simulink model "ImSimulazione"  (Simulink 8.7)
settings: Solver=ode45  StartTime=0.0  StopTime=t(end)+Tf  FixedStep=Tf  RelTol=1e-3
PreLoadFcn:
  | initFunction
InitFcn:
  | initFunctionIm
StopFcn:
  | figure
  | subplot(31,1)
  | plot(err_q.data(1:50))
  | subplot(312)
  | plot(err_dq.data(1:50))
  | subplot(313)
  | plot(err_ddq.data(1:50))
values from neighbouring files (symbols this model uses):
  FM = Kr^-1*Fv*Kr^-1    [ControlloreUnico.m]    (also in SimulazioneLsim.m = Kr^-1*Fv_att*Kr^-1; initFunction.m; initFunctionIm.m)
  Im = Kr^-1*Bconst*Kr^-1    [initFunction.m]    (also in initFunctionIm.m)
  KCA = diag([(-W(1,1)^2 + KM(1,1)*XR(1,1))/(KM(1,1)*KTA(1,1)*W(1,1)^2),             (-W(2,2)^2 + KM(2,2)*XR(2,2))/(KM(2,2)*KTA(2,2)*W(2,2)^2),             (-W(3,3)^2 + KM(3,3)*XR(3,3))/(KM(3,3)*KTA(3,3)*W(3,3)^2),             (-W(4,4)^2 + KM(4,4)*XR(4,4))/(KM(4,4)*KTA(4,4)*W(4,4)^2),             (-W(5,5)^2 + KM(5,5)*XR(5,5))/(KM(5,5)*KTA(5,5)*W(5,5)^2),             (-W(6,6)^2 + KM(6,6)*XR(6,6))/(KM(6,6)* ...(+20 chars)    [DesignControllersAcceleration_6.m]    (also in DesignControllersAcceleration_7.m; DiscreteControllersAcceleration_7.m)
  KM = Kv^-1    [DesignControllersAcceleration_6.m]    (also in DesignControllersAcceleration_7.m; DesignControllersVelocity_6.m; DiscreteControllersAcceleration_7.m; DiscreteDesignControllersVelocity_6.m)
  KTA = diag([100 1 1 1 1 1])    [DesignControllersAcceleration_6.m]    (also in DesignControllersAcceleration_7.m = diag([1 1 1 1 1 1]); DiscreteControllersAcceleration_7.m = diag([1 1 1 1 1 1]))
  KTP = diag([9 1 1 1 1 1])    [DesignControllersAcceleration_6.m]    (also in DesignControllersAcceleration_7.m = diag([1 1 1 1 1 1]); DesignControllersVelocity_6.m = diag([1 1 1 1 1 1]); DiscreteControllersAcceleration_7.m = diag([1 1 1 1 1 1]); DiscreteDesignControllersVelocity_6.m = diag([1 1 1 1 1 1]))
  KTV = diag([4 1 1 1 1 1])    [DesignControllersAcceleration_6.m]    (also in DesignControllersAcceleration_7.m = diag([1 1 1 1 1 1]); DesignControllersVelocity_6.m = diag([1 1 1 1 1 1]); DiscreteControllersAcceleration_7.m = diag([1 1 1 1 1 1]); DiscreteDesignControllersVelocity_6.m = diag([1 1 1 1 1 1]))
  q0 = q0'    [initFunction.m]    (also in initFunctionIm.m)
  T = 0.05    [ComputeBconst_4.m]    (also in ControlloreUnico.m = 0.002; Identificazione_2.m = 0:1/F:(size(min_value,2)-1)*interval; Simulazione.m = 0.002; SimulazioneLsim.m = 0.002)
  Tf = 1/500    (= 0.002)    [ControlloreUnico.m]    (also in Simulazione.m; SimulazioneLsim.m; initFunction.m; initFunctionIm.m)
undefined symbols (not defined in the file or in its folder): gD, gI, gP, Kr, Kt, Kv, La, Ra
libraries: simulink x6
CloseFcn:
  | rtwprivate ssgencode ModelCloseRequest ContributiCoppieComau
settings Model: Creator=Alessandro  LastModifiedBy=Gianluigi  ExtModeAutoUpdateStatusClock=off
settings DataIOCC: SaveFormat=StructureWithTime
settings OptimizationCC: BlockReduction=off  BufferReuse=off  ExpressionDepthLimit=2147483647  InitFltsAndDblsToZero=on
settings DebuggingCC: AlgebraicLoopMsg=none  SaveWithParameterizedLinksMsg=none  SignalResolutionControl=TryResolveAllWithWarning  InheritedTsInSrcMsg=none  MultiTaskDSMMsg=warning  MultiTaskCondExecSysMsg=none  TasksWithSamePriorityMsg=none  FcnCallInpInsideContextMsg=UseLocalSettings  UnconnectedInputMsg=none  UnconnectedOutputMsg=none  UnconnectedLineMsg=none  StateNameClashWarn=warning
settings GRTTargetCC: TargetFcnLib=ansi_tfl_tmw.mat  CombineOutputUpdateFcns=off  GRTInterface=on

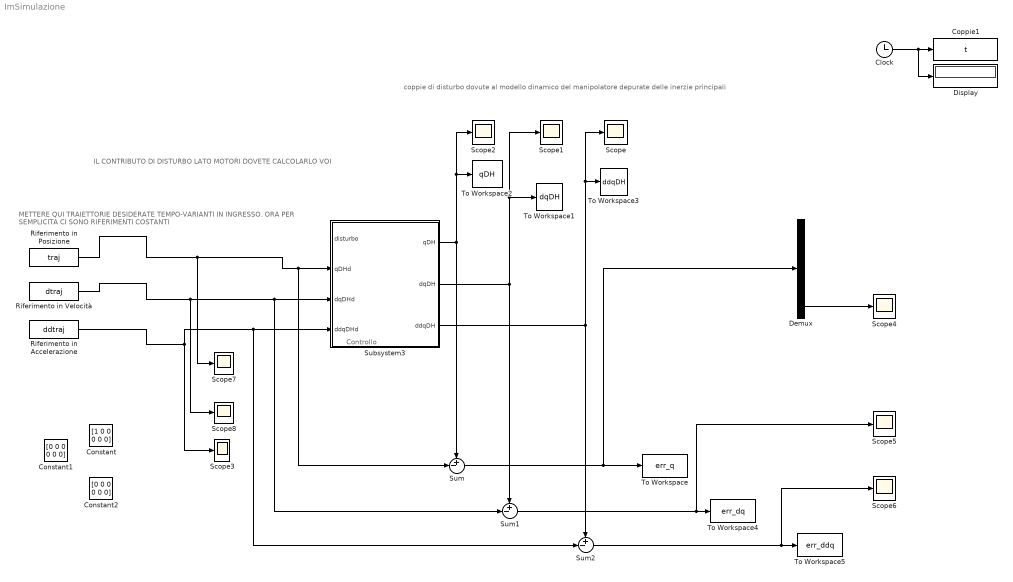
== system ImSimulazione ==
  note: coppie di disturbo dovute al modello dinamico del manipolatore depurate delle inerzie principali
  note: Controllo
  note: METTERE QUI TRAIETTORIE DESIDERATE TEMPO-VARIANTI IN INGRESSO.
      | ORA PER SEMPLICITA CI SONO RIFERIMENTI COSTANTI
  note: IL CONTRIBUTO DI DISTURBO LATO MOTORI DOVETE CALCOLARLO VOI
  Clock : Clock
  Constant : Constant  Value=[1 0 0 0 0 0]
  Constant1 : Constant  Value=[0 0 0 0 0 0]
  Constant2 : Constant  Value=[0 0 0 0 0 0]
  Coppie1 : ToWorkspace  VariableName=t  SampleTime=-1
  Demux : Demux  Outputs=6
  Display : Display
  Riferimento in Accelerazione : FromWorkspace  VariableName=ddtraj
  Riferimento in Posizione : FromWorkspace  VariableName=traj
  Riferimento in Velocità : FromWorkspace  VariableName=dtraj
  Scope{,1..8} (9 alike) : Scope
  Subsystem3 : Subsystem
      mask Display:
      | disp('Controllo');
      | port_label('input', 1, 'disturbo');
      | port_label('input', 2, 'qDHd');
      | port_label('input', 3, 'dqDHd');
      | port_label('output', 1, 'qDH');
      | port_label('output', 2, 'dqDH');
      | port_label('output', 3, 'ddqDH');
  Sum : Sum  Inputs=+-|
  Sum1 : Sum  Inputs=+-|
  Sum2 : Sum  Inputs=+-|
  To Workspace : ToWorkspace  VariableName=err_q  SaveFormat=Timeseries  SampleTime=-1
  To Workspace1 : ToWorkspace  VariableName=dqDH  SampleTime=-1
  To Workspace2 : ToWorkspace  VariableName=qDH  SampleTime=-1
  To Workspace3 : ToWorkspace  VariableName=ddqDH  SampleTime=-1
  To Workspace4 : ToWorkspace  VariableName=err_dq  SaveFormat=Timeseries  SampleTime=-1
  To Workspace5 : ToWorkspace  VariableName=err_ddq  SaveFormat=Timeseries  SampleTime=-1
  wires:
  Clock/1 -> Coppie1/1, Display/1
  Subsystem3/2(dqDH) -> Sum1/1, To Workspace1/1, Scope1/1
  Subsystem3/1(qDH) -> To Workspace2/1, Scope2/1, Sum/1
  Subsystem3/3(ddqDH) -> Sum2/1, To Workspace3/1, Scope/1
  Riferimento in Velocità/1 -> Scope8/1, Sum1/2, Subsystem3/3(dqDHd)
  Riferimento in Accelerazione/1 -> Scope3/1, Sum2/2, Subsystem3/4(ddqDHd)
  Riferimento in Posizione/1 -> Scope7/1, Sum/2, Subsystem3/2(qDHd)
  Sum/1 -> Demux/1, To Workspace/1
  Sum1/1 -> Scope5/1, To Workspace4/1
  Sum2/1 -> Scope6/1, To Workspace5/1
  Demux/6 -> Scope4/1

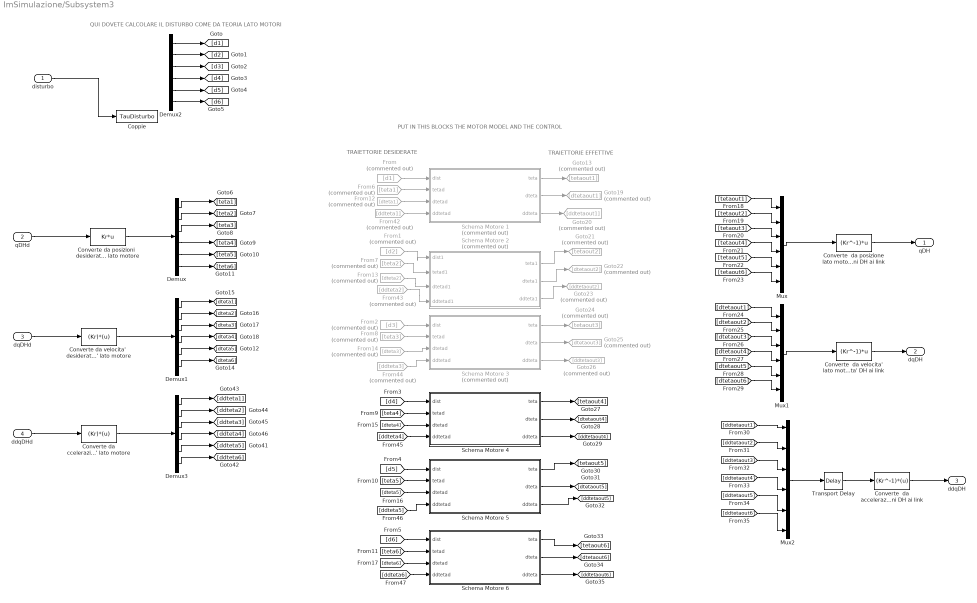
== system ImSimulazione/Subsystem3 ==
  note: PUT IN THIS BLOCKS THE MOTOR MODEL AND THE CONTROL
  note: TRAIETTORIE DESIDERATE
  note: TRAIETTORIE EFFETTIVE
  note: QUI DOVETE CALCOLARE IL DISTURBO COME DA TEORIA LATO MOTORI
  disturbo : Inport
  qDHd : Inport  Port=2
  dqDHd : Inport  Port=3
  ddqDHd : Inport  Port=4
  Converte  da accelerazioni lato motore  ad accelerazioni DH ai link : MATLABFcn  MATLABFcn=(Kr^-1)*(u)
  "Converte  da posizione lato motore a  posizioni DH ai link " : MATLABFcn  MATLABFcn=(Kr^-1)*u
  "Converte  da velocita' lato motore  a velocita' DH ai link " : MATLABFcn  MATLABFcn=(Kr^-1)*u
  Converte da ccelerazioni  desiderate DH ai link  in velocita' lato motore : MATLABFcn  MATLABFcn=(Kr)*(u)
  "Converte da posizioni  desiderate DH ai link  in posizione lato motore " : MATLABFcn  MATLABFcn=Kr*u
  "Converte da velocita'  desiderate DH ai link  in velocita' lato motore " : MATLABFcn  MATLABFcn=(Kr)*(u)
  Coppie : ToWorkspace  VariableName=TauDisturbo  SampleTime=-1
  Demux{,1..3} (4 alike) : Demux  Outputs=6
  From : From  Commented=on  GotoTag=d1
  From1 : From  Commented=on  GotoTag=d2
  From12 : From  Commented=on  GotoTag=dteta1
  From13 : From  Commented=on  GotoTag=dteta2
  From14 : From  Commented=on  GotoTag=dteta3
  From2 : From  Commented=on  GotoTag=d3
  From42 : From  Commented=on  GotoTag=ddteta1
  From43 : From  Commented=on  GotoTag=ddteta2
  From44 : From  Commented=on  GotoTag=ddteta3
  From6 : From  Commented=on  GotoTag=teta1
  From7 : From  Commented=on  GotoTag=teta2
  From8 : From  Commented=on  GotoTag=teta3
  Goto13 : Goto  Commented=on  GotoTag=tetaout1
  Goto19 : Goto  Commented=on  GotoTag=dtetaout1
  Goto20 : Goto  Commented=on  GotoTag=ddtetaout1
  Goto21 : Goto  Commented=on  GotoTag=tetaout2
  Goto22 : Goto  Commented=on  GotoTag=dtetaout2
  Goto23 : Goto  Commented=on  GotoTag=ddtetaout2
  Goto24 : Goto  Commented=on  GotoTag=tetaout3
  Goto25 : Goto  Commented=on  GotoTag=dtetaout3
  Goto26 : Goto  Commented=on  GotoTag=ddtetaout3
  Mux : Mux  Inputs=6
  Mux1 : Mux  Inputs=6
  Mux2 : Mux  Inputs=6
  Schema Motore 1 : Subsystem  Commented=on  mask{i=1}
  Schema Motore 2 : Subsystem  Commented=on  mask{i=2}
  Schema Motore 3 : Subsystem  Commented=on  mask{i=3}
  Schema Motore 4 : Subsystem  mask{i=4}
  Schema Motore 5 : Subsystem  mask{i=5}
  Schema Motore 6 : Subsystem  mask{i=6}
  Transport Delay : TransportDelay  DelayTime=T
  qDH : Outport
  dqDH : Outport  Port=2
  ddqDH : Outport  Port=3
  wires:
  qDHd/1 -> "Converte da posizioni  desiderate DH ai link  in posizione lato motore "/1
  dqDHd/1 -> "Converte da velocita'  desiderate DH ai link  in velocita' lato motore "/1
  "Converte  da velocita' lato motore  a velocita' DH ai link "/1 -> dqDH/1
  Converte  da accelerazioni lato motore  ad accelerazioni DH ai link/1 -> ddqDH/1
  "Converte da posizioni  desiderate DH ai link  in posizione lato motore "/1 -> Demux/1
  disturbo/1 -> Coppie/1
  "Converte  da posizione lato motore a  posizioni DH ai link "/1 -> qDH/1
  Mux/1 -> "Converte  da posizione lato motore a  posizioni DH ai link "/1
  Demux2/1 -> [d1]
  Demux2/2 -> [d2]
  Demux2/3 -> [d3]
  Demux2/4 -> [d4]
  Demux2/5 -> [d5]
  Demux2/6 -> [d6]
  From2/1 -> Schema Motore 3/1(dist)
  [d4] -> Schema Motore 4/1(dist)
  [d5] -> Schema Motore 5/1(dist)
  [d6] -> Schema Motore 6/1(dist)
  Demux/1 -> [teta1]
  Demux/2 -> [teta2]
  Demux/3 -> [teta3]
  Demux/4 -> [teta4]
  Demux/5 -> [teta5]
  Demux/6 -> [teta6]
  From8/1 -> Schema Motore 3/2(tetad)
  [teta4] -> Schema Motore 4/2(tetad)
  [teta5] -> Schema Motore 5/2(tetad)
  [teta6] -> Schema Motore 6/2(tetad)
  "Converte da velocita'  desiderate DH ai link  in velocita' lato motore "/1 -> Demux1/1
  Demux1/1 -> [dteta1]
  Demux1/2 -> [dteta2]
  Demux1/3 -> [dteta3]
  Demux1/4 -> [dteta4]
  Demux1/5 -> [dteta5]
  Demux1/6 -> [dteta6]
  From14/1 -> Schema Motore 3/3(dtetad)
  [dteta4] -> Schema Motore 4/3(dtetad)
  [dteta5] -> Schema Motore 5/3(dtetad)
  [dteta6] -> Schema Motore 6/3(dtetad)
  [tetaout1] -> Mux/1
  [tetaout2] -> Mux/2
  [tetaout3] -> Mux/3
  [tetaout4] -> Mux/4
  [tetaout5] -> Mux/5
  [tetaout6] -> Mux/6
  Mux1/1 -> "Converte  da velocita' lato motore  a velocita' DH ai link "/1
  [dtetaout1] -> Mux1/1
  [dtetaout2] -> Mux1/2
  [dtetaout3] -> Mux1/3
  [dtetaout4] -> Mux1/4
  [dtetaout5] -> Mux1/5
  [dtetaout6] -> Mux1/6
  [ddtetaout1] -> Mux2/1
  [ddtetaout2] -> Mux2/2
  [ddtetaout3] -> Mux2/3
  [ddtetaout4] -> Mux2/4
  [ddtetaout5] -> Mux2/5
  [ddtetaout6] -> Mux2/6
  From6/1 -> Schema Motore 1/2(tetad)
  From12/1 -> Schema Motore 1/3(dtetad)
  Schema Motore 1/1(teta) -> Goto13/1
  Schema Motore 1/2(dteta) -> Goto19/1
  Schema Motore 1/3(ddteta) -> Goto20/1
  From/1 -> Schema Motore 1/1(dist)
  ddqDHd/1 -> Converte da ccelerazioni  desiderate DH ai link  in velocita' lato motore/1
  Demux3/1 -> [ddteta1]
  Demux3/2 -> [ddteta2]
  Demux3/3 -> [ddteta3]
  Demux3/4 -> [ddteta4]
  Demux3/5 -> [ddteta5]
  Demux3/6 -> [ddteta6]
  Converte da ccelerazioni  desiderate DH ai link  in velocita' lato motore/1 -> Demux3/1
  From42/1 -> Schema Motore 1/4(ddtetad)
  Schema Motore 3/1(teta) -> Goto24/1
  Schema Motore 3/2(dteta) -> Goto25/1
  Schema Motore 3/3(ddteta) -> Goto26/1
  Schema Motore 4/1(teta) -> [tetaout4]
  Schema Motore 4/2(dteta) -> [dtetaout4]
  Schema Motore 4/3(ddteta) -> [ddtetaout4]
  Schema Motore 5/1(teta) -> [tetaout5]
  Schema Motore 5/2(dteta) -> [dtetaout5]
  Schema Motore 5/3(ddteta) -> [ddtetaout5]
  Schema Motore 6/1(teta) -> [tetaout6]
  Schema Motore 6/2(dteta) -> [dtetaout6]
  Schema Motore 6/3(ddteta) -> [ddtetaout6]
  From44/1 -> Schema Motore 3/4(ddtetad)
  [ddteta4] -> Schema Motore 4/4(ddtetad)
  [ddteta5] -> Schema Motore 5/4(ddtetad)
  [ddteta6] -> Schema Motore 6/4(ddtetad)
  From1/1 -> Schema Motore 2/1(dist1)
  From7/1 -> Schema Motore 2/2(tetad1)
  From13/1 -> Schema Motore 2/3(dtetad1)
  From43/1 -> Schema Motore 2/4(ddtetad1)
  Schema Motore 2/1(teta1) -> Goto21/1
  Schema Motore 2/2(dteta1) -> Goto22/1
  Schema Motore 2/3(ddteta1) -> Goto23/1
  Mux2/1 -> Transport Delay/1
  Transport Delay/1 -> Converte  da accelerazioni lato motore  ad accelerazioni DH ai link/1

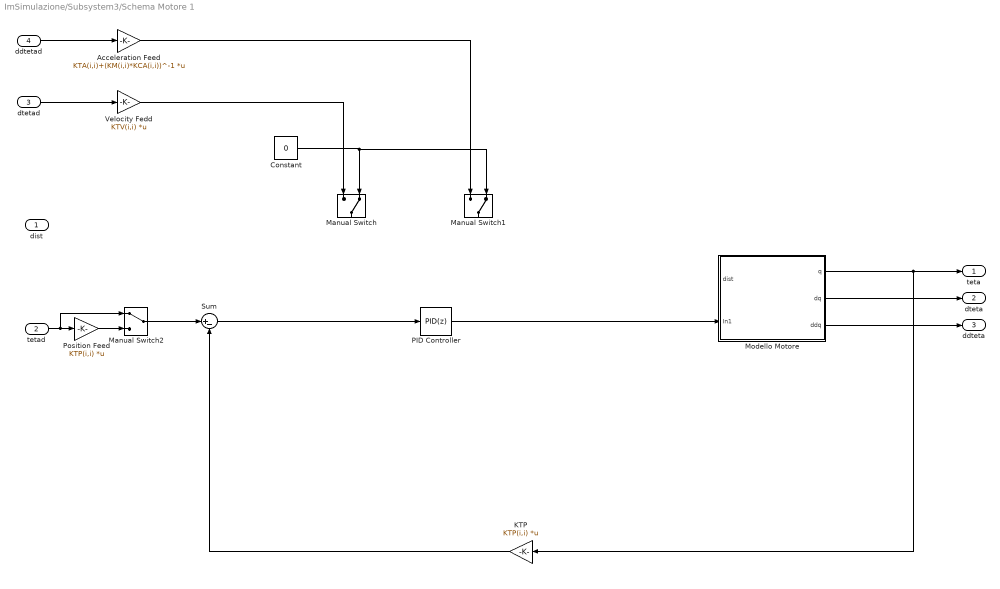
== system ImSimulazione/Subsystem3/Schema Motore 1 ==
  dist : Inport  PortDimensions=1
  tetad : Inport  Port=2  PortDimensions=1
  dtetad : Inport  Port=3  PortDimensions=1
  ddtetad : Inport  Port=4  PortDimensions=1
  Acceleration Feed : Gain  Gain=KTA(i,i)+(KM(i,i)*KCA(i,i))^-1  Multiplication=Matrix(K*u)
  Constant : Constant  Value=0
  KTP : Gain  Gain=KTP(i,i)  Multiplication=Matrix(K*u)
  Manual Switch : ManualSwitch  CurrentSetting=0
  Manual Switch1 : ManualSwitch  CurrentSetting=0
  Manual Switch2 : ManualSwitch
  Modello Motore : Subsystem
  PID Controller : simulink/Continuous/PID Controller  Controller=PID  TimeDomain=Discrete-time  SampleTime=Tf  IntegratorMethod=Forward Euler  FilterMethod=Forward Euler  Form=Parallel  UseFilter=on  ControllerParametersSource=internal  P=gP(i)  I=gI(i)  D=gD(i)  N=100  InitialConditionSource=internal  InitialConditionForIntegrator=0  InitialConditionForFilter=0  ExternalReset=none  LimitOutput=off  UpperSaturationLimit=inf  LowerSaturationLimit=-inf  LinearizeAsGain=on  AntiWindupMode=none  Kb=1  TrackingMode=off  Kt=1  PParamMin=[]  PParamMax=[]  IParamMin=[]  IParamMax=[]  DParamMin=[]  DParamMax=[]  NParamMin=[]  NParamMax=[]  KbParamMin=[]  KbParamMax=[]  KtParamMin=[]  KtParamMax=[]  POutMin=[]  POutMax=[]  IOutMin=[]  IOutMax=[]  DOutMin=[]  DOutMax=[]  NOutMin=[]  NOutMax=[]  KbOutMin=[]  KbOutMax=[]  KtOutMin=[]  KtOutMax=[]  IntegratorOutMin=[]  IntegratorOutMax=[]  FilterOutMin=[]  FilterOutMax=[]  SumOutMin=[]  SumOutMax=[]  SumI1OutMin=[]  SumI1OutMax=[]  SumI2OutMin=[]  SumI2OutMax=[]  SumI3OutMin=[]  SumI3OutMax=[]  SumDOutMin=[]  SumDOutMax=[]  SaturationOutMin=[]  SaturationOutMax=[]  IntegratorContinuousStateAttributes=''  IntegratorStateMustResolveToSignalObject=off  IntegratorRTWStateStorageClass=Auto  FilterContinuousStateAttributes=''  FilterStateMustResolveToSignalObject=off  FilterRTWStateStorageClass=Auto  DifferentiatorICPrevScaledInput=0  DifferentiatorOutMin=[]  DifferentiatorOutMax=[]
  Position Feed : Gain  Gain=KTP(i,i)  Multiplication=Matrix(K*u)
  Sum : Sum  Inputs=|+-
  Velocity Fedd : Gain  Gain=KTV(i,i)  Multiplication=Matrix(K*u)
  teta : Outport  PortDimensions=1
  dteta : Outport  Port=2  PortDimensions=1
  ddteta : Outport  Port=3  PortDimensions=1
  wires:
  Sum/1 -> PID Controller/1
  ddtetad/1 -> Acceleration Feed/1
  KTP/1 -> Sum/2
  Modello Motore/2(dq) -> dteta/1
  Modello Motore/1(q) -> KTP/1, teta/1
  Modello Motore/3(ddq) -> ddteta/1
  dtetad/1 -> Velocity Fedd/1
  Constant/1 -> Manual Switch1/2, Manual Switch/2
  tetad/1 -> Manual Switch2/1, Position Feed/1
  Manual Switch2/1 -> Sum/1
  Position Feed/1 -> Manual Switch2/2
  Velocity Fedd/1 -> Manual Switch/1
  Acceleration Feed/1 -> Manual Switch1/1
  PID Controller/1 -> Modello Motore/2(In1)

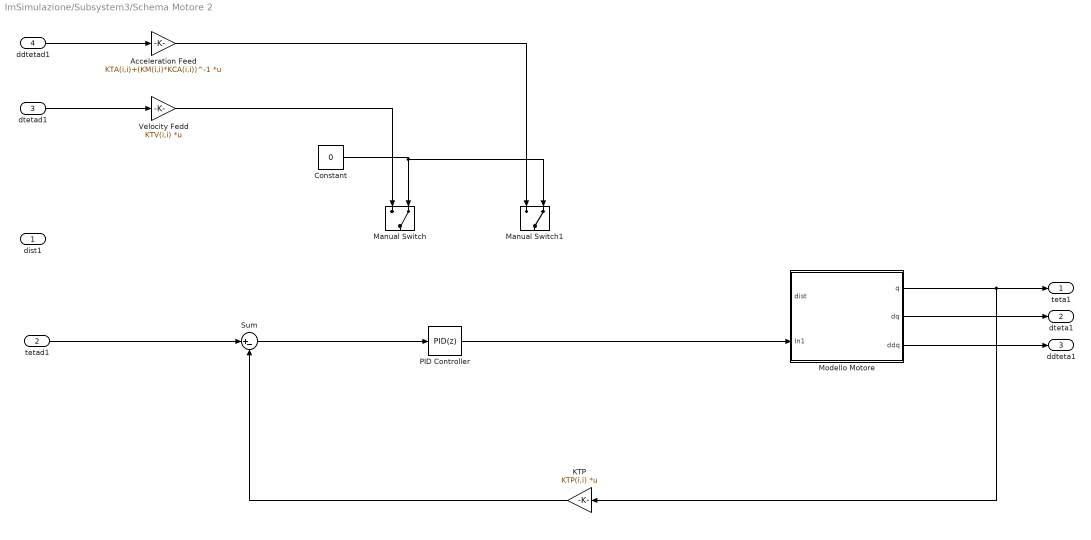
== system ImSimulazione/Subsystem3/Schema Motore 2 ==
  dist1 : Inport  PortDimensions=1
  tetad1 : Inport  Port=2  PortDimensions=1
  dtetad1 : Inport  Port=3  PortDimensions=1
  ddtetad1 : Inport  Port=4  PortDimensions=1
  Acceleration Feed : Gain  Gain=KTA(i,i)+(KM(i,i)*KCA(i,i))^-1  Multiplication=Matrix(K*u)
  Constant : Constant  Value=0
  KTP : Gain  Gain=KTP(i,i)  Multiplication=Matrix(K*u)
  Manual Switch : ManualSwitch  CurrentSetting=0
  Manual Switch1 : ManualSwitch  CurrentSetting=0
  Modello Motore : Subsystem
  PID Controller : simulink/Continuous/PID Controller  Controller=PID  TimeDomain=Discrete-time  SampleTime=Tf  IntegratorMethod=Forward Euler  FilterMethod=Forward Euler  Form=Parallel  UseFilter=on  ControllerParametersSource=internal  P=gP(i)  I=gI(i)  D=gD(i)  N=100  InitialConditionSource=internal  InitialConditionForIntegrator=0  InitialConditionForFilter=0  ExternalReset=none  LimitOutput=off  UpperSaturationLimit=inf  LowerSaturationLimit=-inf  LinearizeAsGain=on  AntiWindupMode=none  Kb=1  TrackingMode=off  Kt=1  PParamMin=[]  PParamMax=[]  IParamMin=[]  IParamMax=[]  DParamMin=[]  DParamMax=[]  NParamMin=[]  NParamMax=[]  KbParamMin=[]  KbParamMax=[]  KtParamMin=[]  KtParamMax=[]  POutMin=[]  POutMax=[]  IOutMin=[]  IOutMax=[]  DOutMin=[]  DOutMax=[]  NOutMin=[]  NOutMax=[]  KbOutMin=[]  KbOutMax=[]  KtOutMin=[]  KtOutMax=[]  IntegratorOutMin=[]  IntegratorOutMax=[]  FilterOutMin=[]  FilterOutMax=[]  SumOutMin=[]  SumOutMax=[]  SumI1OutMin=[]  SumI1OutMax=[]  SumI2OutMin=[]  SumI2OutMax=[]  SumI3OutMin=[]  SumI3OutMax=[]  SumDOutMin=[]  SumDOutMax=[]  SaturationOutMin=[]  SaturationOutMax=[]  IntegratorContinuousStateAttributes=''  IntegratorStateMustResolveToSignalObject=off  IntegratorRTWStateStorageClass=Auto  FilterContinuousStateAttributes=''  FilterStateMustResolveToSignalObject=off  FilterRTWStateStorageClass=Auto  DifferentiatorICPrevScaledInput=0  DifferentiatorOutMin=[]  DifferentiatorOutMax=[]
  Sum : Sum  Inputs=|+-
  Velocity Fedd : Gain  Gain=KTV(i,i)  Multiplication=Matrix(K*u)
  teta1 : Outport  PortDimensions=1
  dteta1 : Outport  Port=2  PortDimensions=1
  ddteta1 : Outport  Port=3  PortDimensions=1
  wires:
  ddtetad1/1 -> Acceleration Feed/1
  KTP/1 -> Sum/2
  Modello Motore/2(dq) -> dteta1/1
  Modello Motore/1(q) -> teta1/1, KTP/1
  Modello Motore/3(ddq) -> ddteta1/1
  dtetad1/1 -> Velocity Fedd/1
  Constant/1 -> Manual Switch1/2, Manual Switch/2
  Velocity Fedd/1 -> Manual Switch/1
  Acceleration Feed/1 -> Manual Switch1/1
  Sum/1 -> PID Controller/1
  PID Controller/1 -> Modello Motore/2(In1)
  tetad1/1 -> Sum/1

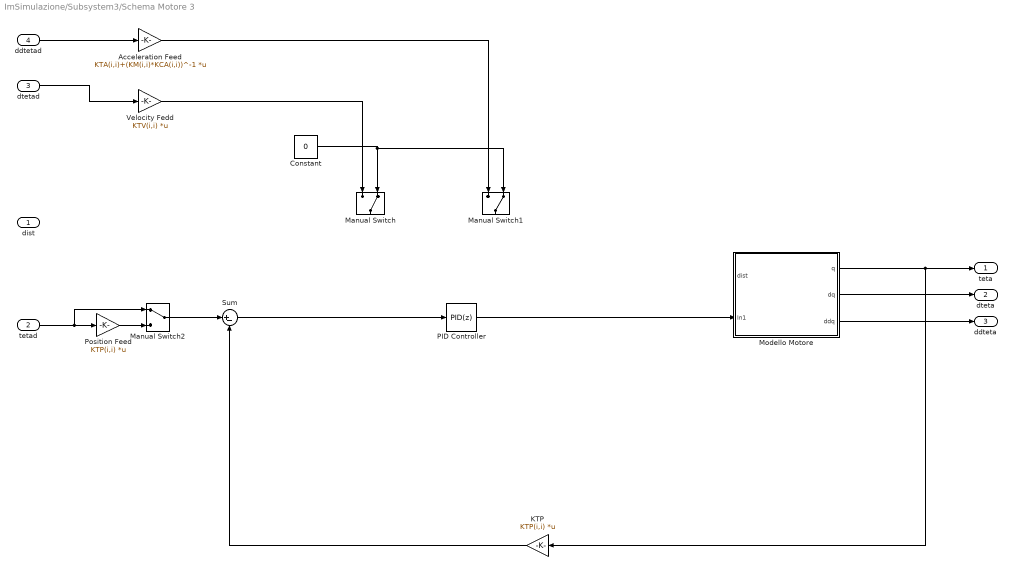
== system ImSimulazione/Subsystem3/Schema Motore 3 ==
  dist : Inport  PortDimensions=1
  tetad : Inport  Port=2  PortDimensions=1
  dtetad : Inport  Port=3  PortDimensions=1
  ddtetad : Inport  Port=4  PortDimensions=1
  Acceleration Feed : Gain  Gain=KTA(i,i)+(KM(i,i)*KCA(i,i))^-1  Multiplication=Matrix(K*u)
  Constant : Constant  Value=0
  KTP : Gain  Gain=KTP(i,i)  Multiplication=Matrix(K*u)
  Manual Switch : ManualSwitch  CurrentSetting=0
  Manual Switch1 : ManualSwitch  CurrentSetting=0
  Manual Switch2 : ManualSwitch
  Modello Motore : Subsystem
  PID Controller : simulink/Continuous/PID Controller  Controller=PID  TimeDomain=Discrete-time  SampleTime=Tf  IntegratorMethod=Forward Euler  FilterMethod=Forward Euler  Form=Parallel  UseFilter=on  ControllerParametersSource=internal  P=gP(i)  I=gI(i)  D=gD(i)  N=100  InitialConditionSource=internal  InitialConditionForIntegrator=0  InitialConditionForFilter=0  ExternalReset=none  LimitOutput=off  UpperSaturationLimit=inf  LowerSaturationLimit=-inf  LinearizeAsGain=on  AntiWindupMode=none  Kb=1  TrackingMode=off  Kt=1  PParamMin=[]  PParamMax=[]  IParamMin=[]  IParamMax=[]  DParamMin=[]  DParamMax=[]  NParamMin=[]  NParamMax=[]  KbParamMin=[]  KbParamMax=[]  KtParamMin=[]  KtParamMax=[]  POutMin=[]  POutMax=[]  IOutMin=[]  IOutMax=[]  DOutMin=[]  DOutMax=[]  NOutMin=[]  NOutMax=[]  KbOutMin=[]  KbOutMax=[]  KtOutMin=[]  KtOutMax=[]  IntegratorOutMin=[]  IntegratorOutMax=[]  FilterOutMin=[]  FilterOutMax=[]  SumOutMin=[]  SumOutMax=[]  SumI1OutMin=[]  SumI1OutMax=[]  SumI2OutMin=[]  SumI2OutMax=[]  SumI3OutMin=[]  SumI3OutMax=[]  SumDOutMin=[]  SumDOutMax=[]  SaturationOutMin=[]  SaturationOutMax=[]  IntegratorContinuousStateAttributes=''  IntegratorStateMustResolveToSignalObject=off  IntegratorRTWStateStorageClass=Auto  FilterContinuousStateAttributes=''  FilterStateMustResolveToSignalObject=off  FilterRTWStateStorageClass=Auto  DifferentiatorICPrevScaledInput=0  DifferentiatorOutMin=[]  DifferentiatorOutMax=[]
  Position Feed : Gain  Gain=KTP(i,i)  Multiplication=Matrix(K*u)
  Sum : Sum  Inputs=|+-
  Velocity Fedd : Gain  Gain=KTV(i,i)  Multiplication=Matrix(K*u)
  teta : Outport  PortDimensions=1
  dteta : Outport  Port=2  PortDimensions=1
  ddteta : Outport  Port=3  PortDimensions=1
  wires:
  ddtetad/1 -> Acceleration Feed/1
  KTP/1 -> Sum/2
  Modello Motore/2(dq) -> dteta/1
  Modello Motore/1(q) -> teta/1, KTP/1
  Modello Motore/3(ddq) -> ddteta/1
  Constant/1 -> Manual Switch1/2, Manual Switch/2
  tetad/1 -> Position Feed/1, Manual Switch2/1
  Manual Switch2/1 -> Sum/1
  Position Feed/1 -> Manual Switch2/2
  Velocity Fedd/1 -> Manual Switch/1
  Acceleration Feed/1 -> Manual Switch1/1
  dtetad/1 -> Velocity Fedd/1
  Sum/1 -> PID Controller/1
  PID Controller/1 -> Modello Motore/2(In1)

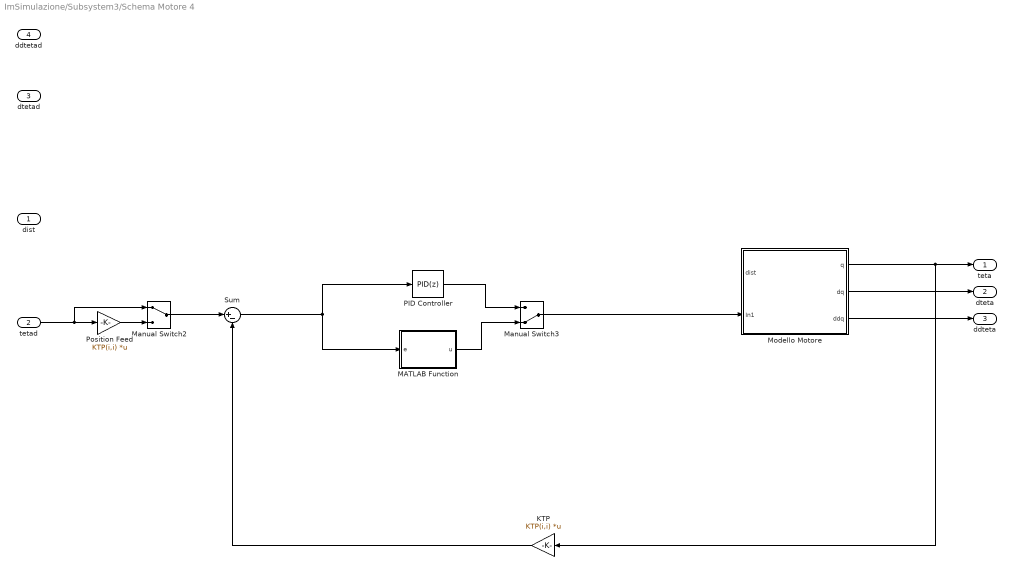
== system ImSimulazione/Subsystem3/Schema Motore 4 ==
  dist : Inport  PortDimensions=1
  tetad : Inport  Port=2  PortDimensions=1
  dtetad : Inport  Port=3  PortDimensions=1
  ddtetad : Inport  Port=4  PortDimensions=1
  KTP : Gain  Gain=KTP(i,i)  Multiplication=Matrix(K*u)
  MATLAB Function : MATLAB Function  TreatAsAtomicUnit=on  SystemSampleTime=Tf
  Manual Switch2 : ManualSwitch
  Manual Switch3 : ManualSwitch  CurrentSetting=0
  Modello Motore : Subsystem
  PID Controller : simulink/Continuous/PID Controller  Controller=PID  TimeDomain=Discrete-time  SampleTime=Tf  IntegratorMethod=Forward Euler  FilterMethod=Forward Euler  Form=Parallel  UseFilter=on  ControllerParametersSource=internal  P=gP(i)  I=gI(i)  D=gD(i)  N=100  InitialConditionSource=internal  InitialConditionForIntegrator=0  InitialConditionForFilter=0  ExternalReset=none  LimitOutput=off  UpperSaturationLimit=inf  LowerSaturationLimit=-inf  LinearizeAsGain=on  AntiWindupMode=none  Kb=1  TrackingMode=off  Kt=1  PParamMin=[]  PParamMax=[]  IParamMin=[]  IParamMax=[]  DParamMin=[]  DParamMax=[]  NParamMin=[]  NParamMax=[]  KbParamMin=[]  KbParamMax=[]  KtParamMin=[]  KtParamMax=[]  POutMin=[]  POutMax=[]  IOutMin=[]  IOutMax=[]  DOutMin=[]  DOutMax=[]  NOutMin=[]  NOutMax=[]  KbOutMin=[]  KbOutMax=[]  KtOutMin=[]  KtOutMax=[]  IntegratorOutMin=[]  IntegratorOutMax=[]  FilterOutMin=[]  FilterOutMax=[]  SumOutMin=[]  SumOutMax=[]  SumI1OutMin=[]  SumI1OutMax=[]  SumI2OutMin=[]  SumI2OutMax=[]  SumI3OutMin=[]  SumI3OutMax=[]  SumDOutMin=[]  SumDOutMax=[]  SaturationOutMin=[]  SaturationOutMax=[]  IntegratorContinuousStateAttributes=''  IntegratorStateMustResolveToSignalObject=off  IntegratorRTWStateStorageClass=Auto  FilterContinuousStateAttributes=''  FilterStateMustResolveToSignalObject=off  FilterRTWStateStorageClass=Auto  DifferentiatorICPrevScaledInput=0  DifferentiatorOutMin=[]  DifferentiatorOutMax=[]
  Position Feed : Gain  Gain=KTP(i,i)  Multiplication=Matrix(K*u)
  Sum : Sum  Inputs=|+-
  teta : Outport  PortDimensions=1
  dteta : Outport  Port=2  PortDimensions=1
  ddteta : Outport  Port=3  PortDimensions=1
  wires:
  KTP/1 -> Sum/2
  Modello Motore/2(dq) -> dteta/1
  Modello Motore/1(q) -> teta/1, KTP/1
  Modello Motore/3(ddq) -> ddteta/1
  tetad/1 -> Position Feed/1, Manual Switch2/1
  Manual Switch2/1 -> Sum/1
  Position Feed/1 -> Manual Switch2/2
  Sum/1 -> MATLAB Function/1(e), PID Controller/1
  Manual Switch3/1 -> Modello Motore/2(In1)
  PID Controller/1 -> Manual Switch3/1
  MATLAB Function/1(u) -> Manual Switch3/2

== system ImSimulazione/Subsystem3/Schema Motore 5 ==
  dist : Inport  PortDimensions=1
  tetad : Inport  Port=2  PortDimensions=1
  dtetad : Inport  Port=3  PortDimensions=1
  ddtetad : Inport  Port=4  PortDimensions=1
  KTP : Gain  Gain=KTP(i,i)  Multiplication=Matrix(K*u)
  MATLAB Function : MATLAB Function  TreatAsAtomicUnit=on  SystemSampleTime=Tf
  Manual Switch2 : ManualSwitch
  Manual Switch3 : ManualSwitch  CurrentSetting=0
  Modello Motore : Subsystem
  PID Controller : simulink/Continuous/PID Controller  Controller=PID  TimeDomain=Discrete-time  SampleTime=Tf  IntegratorMethod=Forward Euler  FilterMethod=Forward Euler  Form=Parallel  UseFilter=on  ControllerParametersSource=internal  P=gP(i)  I=gI(i)  D=gD(i)  N=100  InitialConditionSource=internal  InitialConditionForIntegrator=0  InitialConditionForFilter=0  ExternalReset=none  LimitOutput=off  UpperSaturationLimit=inf  LowerSaturationLimit=-inf  LinearizeAsGain=on  AntiWindupMode=none  Kb=1  TrackingMode=off  Kt=1  PParamMin=[]  PParamMax=[]  IParamMin=[]  IParamMax=[]  DParamMin=[]  DParamMax=[]  NParamMin=[]  NParamMax=[]  KbParamMin=[]  KbParamMax=[]  KtParamMin=[]  KtParamMax=[]  POutMin=[]  POutMax=[]  IOutMin=[]  IOutMax=[]  DOutMin=[]  DOutMax=[]  NOutMin=[]  NOutMax=[]  KbOutMin=[]  KbOutMax=[]  KtOutMin=[]  KtOutMax=[]  IntegratorOutMin=[]  IntegratorOutMax=[]  FilterOutMin=[]  FilterOutMax=[]  SumOutMin=[]  SumOutMax=[]  SumI1OutMin=[]  SumI1OutMax=[]  SumI2OutMin=[]  SumI2OutMax=[]  SumI3OutMin=[]  SumI3OutMax=[]  SumDOutMin=[]  SumDOutMax=[]  SaturationOutMin=[]  SaturationOutMax=[]  IntegratorContinuousStateAttributes=''  IntegratorStateMustResolveToSignalObject=off  IntegratorRTWStateStorageClass=Auto  FilterContinuousStateAttributes=''  FilterStateMustResolveToSignalObject=off  FilterRTWStateStorageClass=Auto  DifferentiatorICPrevScaledInput=0  DifferentiatorOutMin=[]  DifferentiatorOutMax=[]
  Position Feed : Gain  Gain=KTP(i,i)  Multiplication=Matrix(K*u)
  Sum : Sum  Inputs=|+-
  teta : Outport  PortDimensions=1
  dteta : Outport  Port=2  PortDimensions=1
  ddteta : Outport  Port=3  PortDimensions=1
  wires:
  KTP/1 -> Sum/2
  Modello Motore/2(dq) -> dteta/1
  Modello Motore/1(q) -> teta/1, KTP/1
  Modello Motore/3(ddq) -> ddteta/1
  tetad/1 -> Position Feed/1, Manual Switch2/1
  Manual Switch2/1 -> Sum/1
  Position Feed/1 -> Manual Switch2/2
  Sum/1 -> MATLAB Function/1(e), PID Controller/1
  Manual Switch3/1 -> Modello Motore/2(In1)
  PID Controller/1 -> Manual Switch3/1
  MATLAB Function/1(u) -> Manual Switch3/2

== system ImSimulazione/Subsystem3/Schema Motore 6 ==
  dist : Inport  PortDimensions=1
  tetad : Inport  Port=2  PortDimensions=1
  dtetad : Inport  Port=3  PortDimensions=1
  ddtetad : Inport  Port=4  PortDimensions=1
  KTP : Gain  Gain=KTP(i,i)  Multiplication=Matrix(K*u)
  MATLAB Function : MATLAB Function  TreatAsAtomicUnit=on  SystemSampleTime=Tf
  Manual Switch2 : ManualSwitch
  Manual Switch3 : ManualSwitch  CurrentSetting=0
  Modello Motore : Subsystem
  PID Controller : simulink/Continuous/PID Controller  Controller=PID  TimeDomain=Discrete-time  SampleTime=Tf  IntegratorMethod=Forward Euler  FilterMethod=Forward Euler  Form=Parallel  UseFilter=on  ControllerParametersSource=internal  P=gP(i)  I=gI(i)  D=gD(i)  N=100  InitialConditionSource=internal  InitialConditionForIntegrator=0  InitialConditionForFilter=0  ExternalReset=none  LimitOutput=off  UpperSaturationLimit=inf  LowerSaturationLimit=-inf  LinearizeAsGain=on  AntiWindupMode=none  Kb=1  TrackingMode=off  Kt=1  PParamMin=[]  PParamMax=[]  IParamMin=[]  IParamMax=[]  DParamMin=[]  DParamMax=[]  NParamMin=[]  NParamMax=[]  KbParamMin=[]  KbParamMax=[]  KtParamMin=[]  KtParamMax=[]  POutMin=[]  POutMax=[]  IOutMin=[]  IOutMax=[]  DOutMin=[]  DOutMax=[]  NOutMin=[]  NOutMax=[]  KbOutMin=[]  KbOutMax=[]  KtOutMin=[]  KtOutMax=[]  IntegratorOutMin=[]  IntegratorOutMax=[]  FilterOutMin=[]  FilterOutMax=[]  SumOutMin=[]  SumOutMax=[]  SumI1OutMin=[]  SumI1OutMax=[]  SumI2OutMin=[]  SumI2OutMax=[]  SumI3OutMin=[]  SumI3OutMax=[]  SumDOutMin=[]  SumDOutMax=[]  SaturationOutMin=[]  SaturationOutMax=[]  IntegratorContinuousStateAttributes=''  IntegratorStateMustResolveToSignalObject=off  IntegratorRTWStateStorageClass=Auto  FilterContinuousStateAttributes=''  FilterStateMustResolveToSignalObject=off  FilterRTWStateStorageClass=Auto  DifferentiatorICPrevScaledInput=0  DifferentiatorOutMin=[]  DifferentiatorOutMax=[]
  Position Feed : Gain  Gain=KTP(i,i)  Multiplication=Matrix(K*u)
  Sum : Sum  Inputs=|+-
  teta : Outport  PortDimensions=1
  dteta : Outport  Port=2  PortDimensions=1
  ddteta : Outport  Port=3  PortDimensions=1
  wires:
  KTP/1 -> Sum/2
  Modello Motore/2(dq) -> dteta/1
  Modello Motore/1(q) -> teta/1, KTP/1
  Modello Motore/3(ddq) -> ddteta/1
  tetad/1 -> Position Feed/1, Manual Switch2/1
  Manual Switch2/1 -> Sum/1
  Position Feed/1 -> Manual Switch2/2
  Sum/1 -> PID Controller/1, MATLAB Function/1(e)
  PID Controller/1 -> Manual Switch3/1
  Manual Switch3/1 -> Modello Motore/2(In1)
  MATLAB Function/1(u) -> Manual Switch3/2

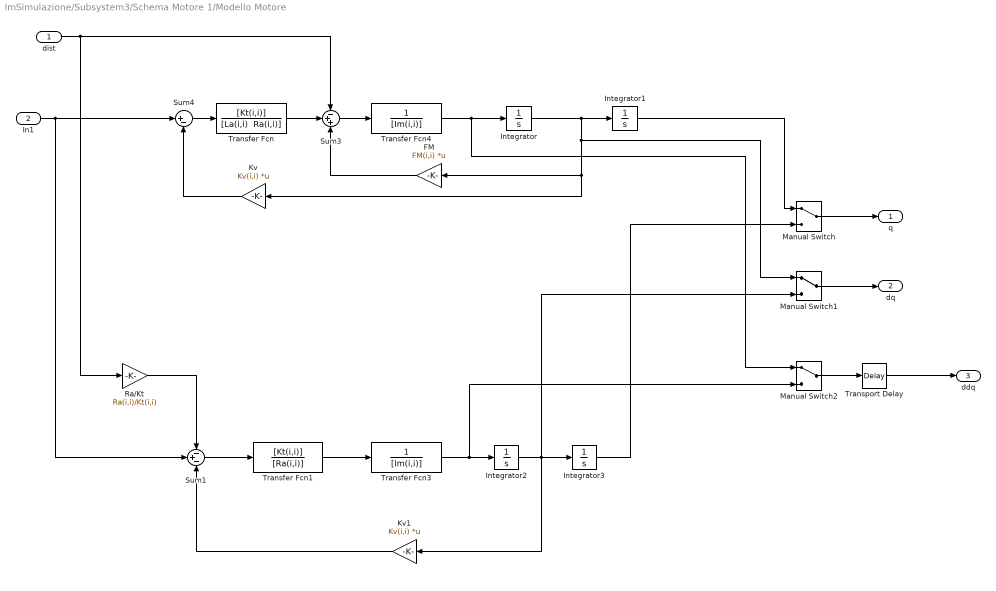
== system ImSimulazione/Subsystem3/Schema Motore 1/Modello Motore ==
  dist : Inport
  In1 : Inport  Port=2
  FM : Gain  Gain=FM(i,i)  Multiplication=Matrix(K*u)
  Integrator : Integrator
  Integrator1 : Integrator  InitialCondition=q0(i)
  Integrator2 : Integrator
  Integrator3 : Integrator  InitialCondition=q0(i)
  Kv : Gain  Gain=Kv(i,i)  Multiplication=Matrix(K*u)
  Kv1 : Gain  Gain=Kv(i,i)  Multiplication=Matrix(K*u)
  Manual Switch : ManualSwitch
  Manual Switch1 : ManualSwitch
  Manual Switch2 : ManualSwitch
  Ra/Kt : Gain  Gain=Ra(i,i)/Kt(i,i)
  Sum1 : Sum  Inputs=-+-
  Sum3 : Sum  Inputs=-++
  Sum4 : Sum  Inputs=|+-
  Transfer Fcn : TransferFcn  Numerator=[Kt(i,i)]  Denominator="[La(i,i)  Ra(i,i)]"
  Transfer Fcn1 : TransferFcn  Numerator=[Kt(i,i)]  Denominator=[Ra(i,i)]
  Transfer Fcn3 : TransferFcn  Denominator=[Im(i,i)]
  Transfer Fcn4 : TransferFcn  Denominator=[Im(i,i)]
  Transport Delay : TransportDelay  DelayTime=0.1*T
  q : Outport
  dq : Outport  Port=2
  ddq : Outport  Port=3
  wires:
  Manual Switch1/1 -> dq/1
  Manual Switch/1 -> q/1
  Integrator/1 -> Kv/1, FM/1, Manual Switch1/1, Integrator1/1
  Kv/1 -> Sum4/2
  In1/1 -> Sum1/2, Sum4/1
  Sum4/1 -> Transfer Fcn/1
  Transfer Fcn/1 -> Sum3/2
  FM/1 -> Sum3/3
  Integrator1/1 -> Manual Switch/1
  dist/1 -> Ra/Kt/1, Sum3/1
  Ra/Kt/1 -> Sum1/1
  Sum1/1 -> Transfer Fcn1/1
  Transfer Fcn1/1 -> Transfer Fcn3/1
  Transfer Fcn3/1 -> Manual Switch2/2, Integrator2/1
  Integrator2/1 -> Manual Switch1/2, Kv1/1, Integrator3/1
  Kv1/1 -> Sum1/3
  Integrator3/1 -> Manual Switch/2
  Sum3/1 -> Transfer Fcn4/1
  Transfer Fcn4/1 -> Manual Switch2/1, Integrator/1
  Manual Switch2/1 -> Transport Delay/1
  Transport Delay/1 -> ddq/1

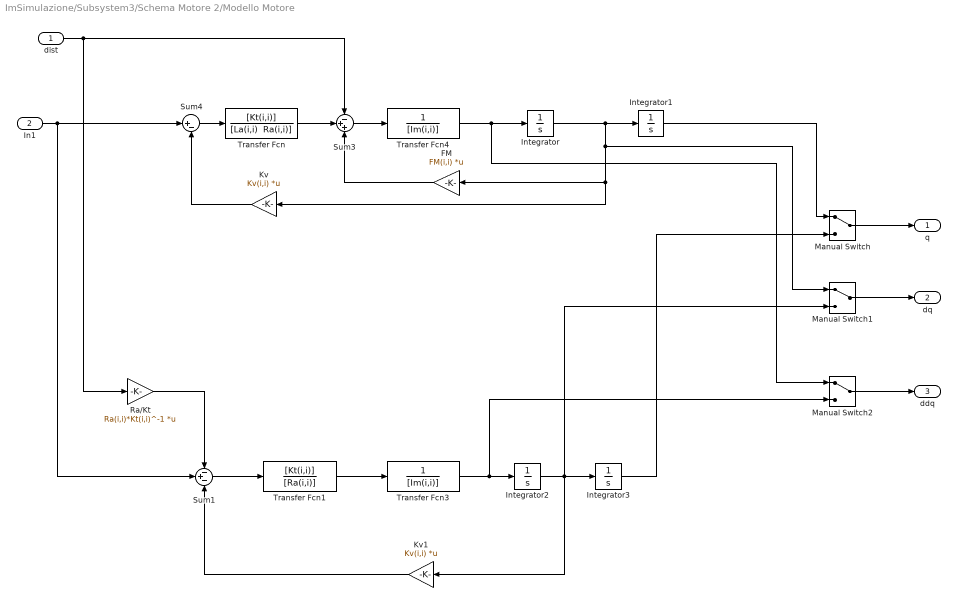
== system ImSimulazione/Subsystem3/Schema Motore 2/Modello Motore ==
  dist : Inport
  In1 : Inport  Port=2
  FM : Gain  Gain=FM(i,i)  Multiplication=Matrix(K*u)
  Integrator : Integrator
  Integrator1 : Integrator  InitialCondition=q0(i)
  Integrator2 : Integrator
  Integrator3 : Integrator  InitialCondition=q0(i)
  Kv : Gain  Gain=Kv(i,i)  Multiplication=Matrix(K*u)
  Kv1 : Gain  Gain=Kv(i,i)  Multiplication=Matrix(K*u)
  Manual Switch : ManualSwitch
  Manual Switch1 : ManualSwitch
  Manual Switch2 : ManualSwitch
  Ra/Kt : Gain  Gain=Ra(i,i)*Kt(i,i)^-1  Multiplication=Matrix(K*u)
  Sum1 : Sum  Inputs=-+-
  Sum3 : Sum  Inputs=-++
  Sum4 : Sum  Inputs=|+-
  Transfer Fcn : TransferFcn  Numerator=[Kt(i,i)]  Denominator="[La(i,i)  Ra(i,i)]"
  Transfer Fcn1 : TransferFcn  Numerator=[Kt(i,i)]  Denominator=[Ra(i,i)]
  Transfer Fcn3 : TransferFcn  Denominator=[Im(i,i)]
  Transfer Fcn4 : TransferFcn  Denominator=[Im(i,i)]
  q : Outport
  dq : Outport  Port=2
  ddq : Outport  Port=3
  wires:
  Manual Switch2/1 -> ddq/1
  Manual Switch1/1 -> dq/1
  Manual Switch/1 -> q/1
  Integrator/1 -> Kv/1, FM/1, Manual Switch1/1, Integrator1/1
  Kv/1 -> Sum4/2
  In1/1 -> Sum1/2, Sum4/1
  Sum4/1 -> Transfer Fcn/1
  Transfer Fcn/1 -> Sum3/2
  FM/1 -> Sum3/3
  Integrator1/1 -> Manual Switch/1
  dist/1 -> Ra/Kt/1, Sum3/1
  Ra/Kt/1 -> Sum1/1
  Sum1/1 -> Transfer Fcn1/1
  Transfer Fcn1/1 -> Transfer Fcn3/1
  Transfer Fcn3/1 -> Manual Switch2/2, Integrator2/1
  Integrator2/1 -> Manual Switch1/2, Kv1/1, Integrator3/1
  Kv1/1 -> Sum1/3
  Integrator3/1 -> Manual Switch/2
  Sum3/1 -> Transfer Fcn4/1
  Transfer Fcn4/1 -> Manual Switch2/1, Integrator/1

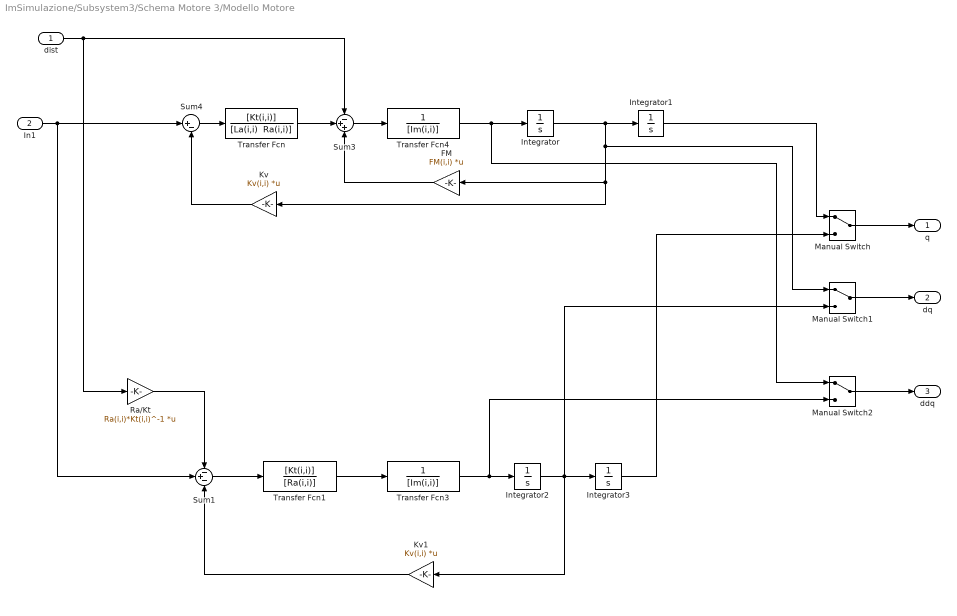
== system ImSimulazione/Subsystem3/Schema Motore 3/Modello Motore ==
  dist : Inport
  In1 : Inport  Port=2
  FM : Gain  Gain=FM(i,i)  Multiplication=Matrix(K*u)
  Integrator : Integrator
  Integrator1 : Integrator  InitialCondition=q0(i)
  Integrator2 : Integrator
  Integrator3 : Integrator  InitialCondition=q0(i)
  Kv : Gain  Gain=Kv(i,i)  Multiplication=Matrix(K*u)
  Kv1 : Gain  Gain=Kv(i,i)  Multiplication=Matrix(K*u)
  Manual Switch : ManualSwitch
  Manual Switch1 : ManualSwitch
  Manual Switch2 : ManualSwitch
  Ra/Kt : Gain  Gain=Ra(i,i)*Kt(i,i)^-1  Multiplication=Matrix(K*u)
  Sum1 : Sum  Inputs=-+-
  Sum3 : Sum  Inputs=-++
  Sum4 : Sum  Inputs=|+-
  Transfer Fcn : TransferFcn  Numerator=[Kt(i,i)]  Denominator="[La(i,i)  Ra(i,i)]"
  Transfer Fcn1 : TransferFcn  Numerator=[Kt(i,i)]  Denominator=[Ra(i,i)]
  Transfer Fcn3 : TransferFcn  Denominator=[Im(i,i)]
  Transfer Fcn4 : TransferFcn  Denominator=[Im(i,i)]
  q : Outport
  dq : Outport  Port=2
  ddq : Outport  Port=3
  wires:
  Manual Switch2/1 -> ddq/1
  Manual Switch1/1 -> dq/1
  Manual Switch/1 -> q/1
  Integrator/1 -> Kv/1, FM/1, Manual Switch1/1, Integrator1/1
  Kv/1 -> Sum4/2
  In1/1 -> Sum1/2, Sum4/1
  Sum4/1 -> Transfer Fcn/1
  Transfer Fcn/1 -> Sum3/2
  FM/1 -> Sum3/3
  Integrator1/1 -> Manual Switch/1
  dist/1 -> Ra/Kt/1, Sum3/1
  Ra/Kt/1 -> Sum1/1
  Sum1/1 -> Transfer Fcn1/1
  Transfer Fcn1/1 -> Transfer Fcn3/1
  Transfer Fcn3/1 -> Manual Switch2/2, Integrator2/1
  Integrator2/1 -> Manual Switch1/2, Kv1/1, Integrator3/1
  Kv1/1 -> Sum1/3
  Integrator3/1 -> Manual Switch/2
  Sum3/1 -> Transfer Fcn4/1
  Transfer Fcn4/1 -> Manual Switch2/1, Integrator/1

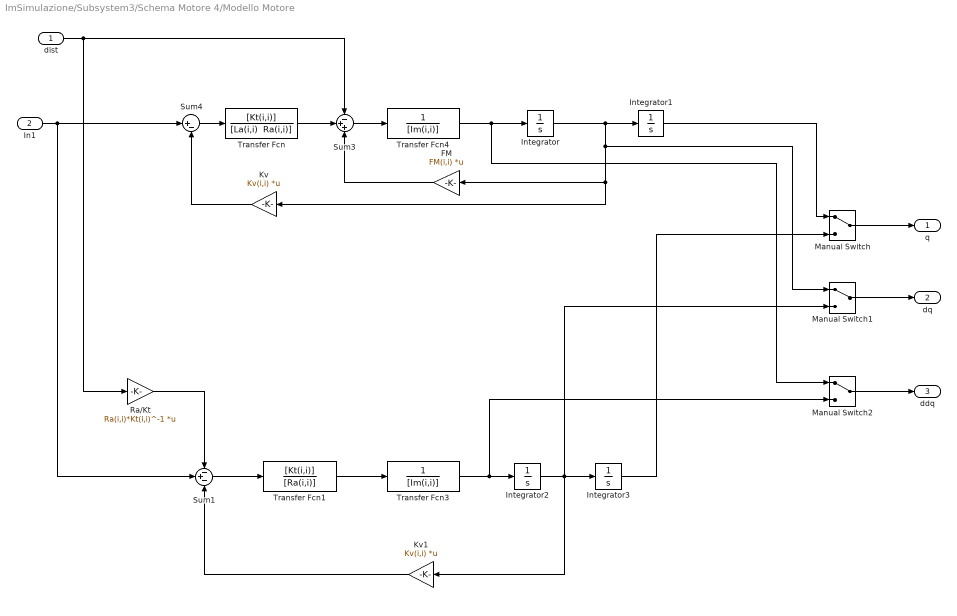
== system ImSimulazione/Subsystem3/Schema Motore 4/Modello Motore ==
  dist : Inport
  In1 : Inport  Port=2
  FM : Gain  Gain=FM(i,i)  Multiplication=Matrix(K*u)
  Integrator : Integrator
  Integrator1 : Integrator  InitialCondition=q0(i)
  Integrator2 : Integrator
  Integrator3 : Integrator  InitialCondition=q0(i)
  Kv : Gain  Gain=Kv(i,i)  Multiplication=Matrix(K*u)
  Kv1 : Gain  Gain=Kv(i,i)  Multiplication=Matrix(K*u)
  Manual Switch : ManualSwitch
  Manual Switch1 : ManualSwitch
  Manual Switch2 : ManualSwitch
  Ra/Kt : Gain  Gain=Ra(i,i)*Kt(i,i)^-1  Multiplication=Matrix(K*u)
  Sum1 : Sum  Inputs=-+-
  Sum3 : Sum  Inputs=-++
  Sum4 : Sum  Inputs=|+-
  Transfer Fcn : TransferFcn  Numerator=[Kt(i,i)]  Denominator="[La(i,i)  Ra(i,i)]"
  Transfer Fcn1 : TransferFcn  Numerator=[Kt(i,i)]  Denominator=[Ra(i,i)]
  Transfer Fcn3 : TransferFcn  Denominator=[Im(i,i)]
  Transfer Fcn4 : TransferFcn  Denominator=[Im(i,i)]
  q : Outport
  dq : Outport  Port=2
  ddq : Outport  Port=3
  wires:
  Manual Switch2/1 -> ddq/1
  Manual Switch1/1 -> dq/1
  Manual Switch/1 -> q/1
  Integrator/1 -> Kv/1, FM/1, Manual Switch1/1, Integrator1/1
  Kv/1 -> Sum4/2
  In1/1 -> Sum1/2, Sum4/1
  Sum4/1 -> Transfer Fcn/1
  Transfer Fcn/1 -> Sum3/2
  FM/1 -> Sum3/3
  Integrator1/1 -> Manual Switch/1
  dist/1 -> Ra/Kt/1, Sum3/1
  Ra/Kt/1 -> Sum1/1
  Sum1/1 -> Transfer Fcn1/1
  Transfer Fcn1/1 -> Transfer Fcn3/1
  Transfer Fcn3/1 -> Manual Switch2/2, Integrator2/1
  Integrator2/1 -> Manual Switch1/2, Kv1/1, Integrator3/1
  Kv1/1 -> Sum1/3
  Integrator3/1 -> Manual Switch/2
  Sum3/1 -> Transfer Fcn4/1
  Transfer Fcn4/1 -> Manual Switch2/1, Integrator/1

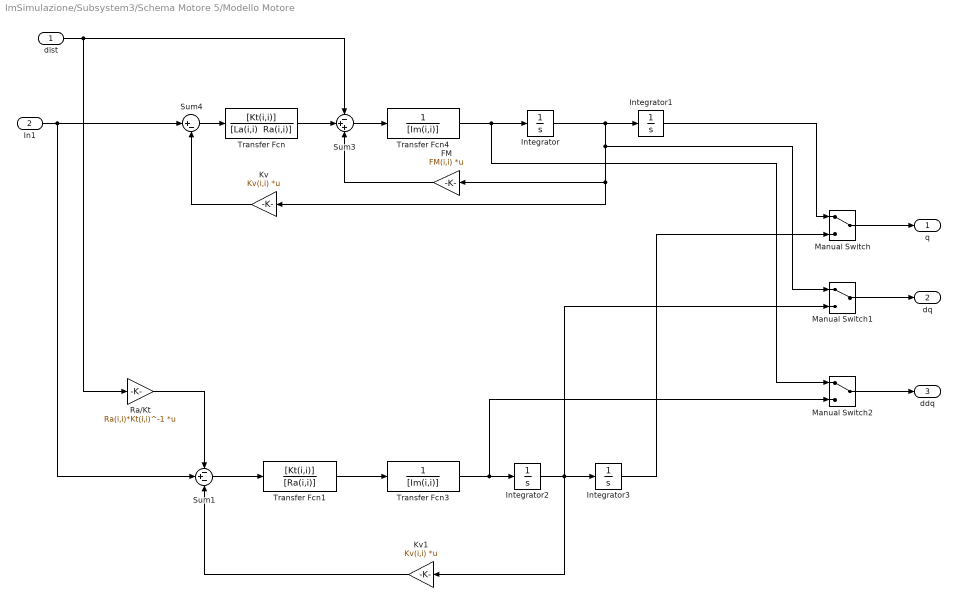
== system ImSimulazione/Subsystem3/Schema Motore 5/Modello Motore ==
  dist : Inport
  In1 : Inport  Port=2
  FM : Gain  Gain=FM(i,i)  Multiplication=Matrix(K*u)
  Integrator : Integrator
  Integrator1 : Integrator  InitialCondition=q0(i)
  Integrator2 : Integrator
  Integrator3 : Integrator  InitialCondition=q0(i)
  Kv : Gain  Gain=Kv(i,i)  Multiplication=Matrix(K*u)
  Kv1 : Gain  Gain=Kv(i,i)  Multiplication=Matrix(K*u)
  Manual Switch : ManualSwitch
  Manual Switch1 : ManualSwitch
  Manual Switch2 : ManualSwitch
  Ra/Kt : Gain  Gain=Ra(i,i)*Kt(i,i)^-1  Multiplication=Matrix(K*u)
  Sum1 : Sum  Inputs=-+-
  Sum3 : Sum  Inputs=-++
  Sum4 : Sum  Inputs=|+-
  Transfer Fcn : TransferFcn  Numerator=[Kt(i,i)]  Denominator="[La(i,i)  Ra(i,i)]"
  Transfer Fcn1 : TransferFcn  Numerator=[Kt(i,i)]  Denominator=[Ra(i,i)]
  Transfer Fcn3 : TransferFcn  Denominator=[Im(i,i)]
  Transfer Fcn4 : TransferFcn  Denominator=[Im(i,i)]
  q : Outport
  dq : Outport  Port=2
  ddq : Outport  Port=3
  wires:
  Manual Switch2/1 -> ddq/1
  Manual Switch1/1 -> dq/1
  Manual Switch/1 -> q/1
  Integrator/1 -> Kv/1, FM/1, Manual Switch1/1, Integrator1/1
  Kv/1 -> Sum4/2
  In1/1 -> Sum1/2, Sum4/1
  Sum4/1 -> Transfer Fcn/1
  Transfer Fcn/1 -> Sum3/2
  FM/1 -> Sum3/3
  Integrator1/1 -> Manual Switch/1
  dist/1 -> Ra/Kt/1, Sum3/1
  Ra/Kt/1 -> Sum1/1
  Sum1/1 -> Transfer Fcn1/1
  Transfer Fcn1/1 -> Transfer Fcn3/1
  Transfer Fcn3/1 -> Manual Switch2/2, Integrator2/1
  Integrator2/1 -> Manual Switch1/2, Kv1/1, Integrator3/1
  Kv1/1 -> Sum1/3
  Integrator3/1 -> Manual Switch/2
  Sum3/1 -> Transfer Fcn4/1
  Transfer Fcn4/1 -> Manual Switch2/1, Integrator/1

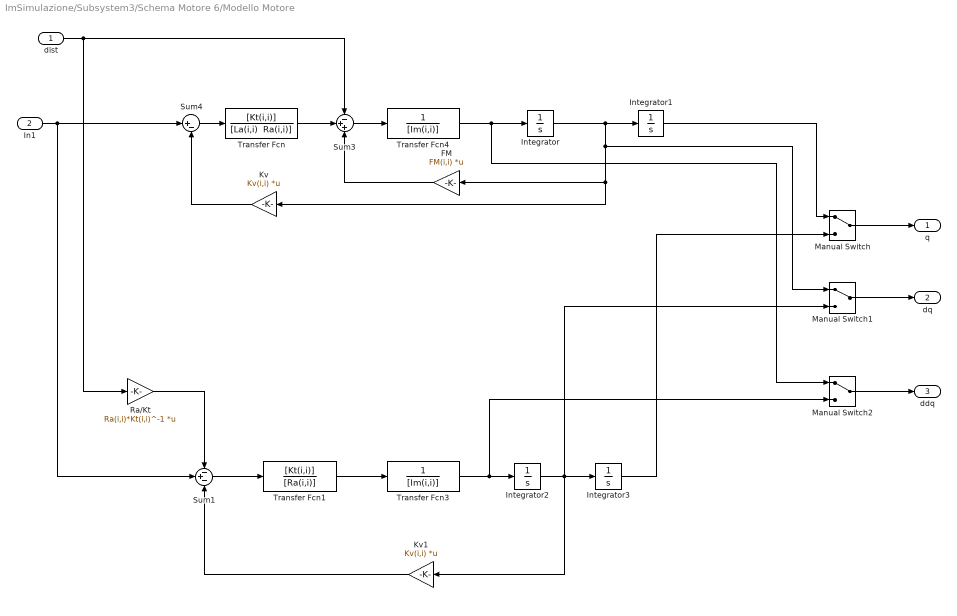
== system ImSimulazione/Subsystem3/Schema Motore 6/Modello Motore ==
  dist : Inport
  In1 : Inport  Port=2
  FM : Gain  Gain=FM(i,i)  Multiplication=Matrix(K*u)
  Integrator : Integrator
  Integrator1 : Integrator  InitialCondition=q0(i)
  Integrator2 : Integrator
  Integrator3 : Integrator  InitialCondition=q0(i)
  Kv : Gain  Gain=Kv(i,i)  Multiplication=Matrix(K*u)
  Kv1 : Gain  Gain=Kv(i,i)  Multiplication=Matrix(K*u)
  Manual Switch : ManualSwitch
  Manual Switch1 : ManualSwitch
  Manual Switch2 : ManualSwitch
  Ra/Kt : Gain  Gain=Ra(i,i)*Kt(i,i)^-1  Multiplication=Matrix(K*u)
  Sum1 : Sum  Inputs=-+-
  Sum3 : Sum  Inputs=-++
  Sum4 : Sum  Inputs=|+-
  Transfer Fcn : TransferFcn  Numerator=[Kt(i,i)]  Denominator="[La(i,i)  Ra(i,i)]"
  Transfer Fcn1 : TransferFcn  Numerator=[Kt(i,i)]  Denominator=[Ra(i,i)]
  Transfer Fcn3 : TransferFcn  Denominator=[Im(i,i)]
  Transfer Fcn4 : TransferFcn  Denominator=[Im(i,i)]
  q : Outport
  dq : Outport  Port=2
  ddq : Outport  Port=3
  wires:
  Manual Switch2/1 -> ddq/1
  Manual Switch1/1 -> dq/1
  Manual Switch/1 -> q/1
  Integrator/1 -> Kv/1, FM/1, Manual Switch1/1, Integrator1/1
  Kv/1 -> Sum4/2
  In1/1 -> Sum1/2, Sum4/1
  Sum4/1 -> Transfer Fcn/1
  Transfer Fcn/1 -> Sum3/2
  FM/1 -> Sum3/3
  Integrator1/1 -> Manual Switch/1
  dist/1 -> Ra/Kt/1, Sum3/1
  Ra/Kt/1 -> Sum1/1
  Sum1/1 -> Transfer Fcn1/1
  Transfer Fcn1/1 -> Transfer Fcn3/1
  Transfer Fcn3/1 -> Manual Switch2/2, Integrator2/1
  Integrator2/1 -> Manual Switch1/2, Kv1/1, Integrator3/1
  Kv1/1 -> Sum1/3
  Integrator3/1 -> Manual Switch/2
  Sum3/1 -> Transfer Fcn4/1
  Transfer Fcn4/1 -> Manual Switch2/1, Integrator/1

== matlab function Subsystem3/Schema Motore 5/MATLAB Function ==
  data: e input double; u output double
function u = fcn(e)
persistent uOld;
persistent uOldOld;
persistent eOld;
persistent eOldOld;
if isempty(uOld)
   uOld = 0;
end
if isempty(uOldOld)
   uOldOld = 0;
end
if isempty(eOld)
   eOld = 0;
end
if isempty(eOldOld)
   eOldOld = 0;
end
%   9328 z^2 - 1.553e04 z + 6464    U(z)
%   ---------------------------- = -----
%        z^2 - 1.8 z + 0.8          E(z)
% U(z)*(z^2 - 1.8 z + 0.8) = E(z)*(9328 z^2 - 1.553e04 z + 6464)
u = 1.8*uOld - 0.8*uOldOld + 9328*e - 15530*eOld + 6464*eOldOld;

uOldOld = uOld;
uOld = u;
eOldOld = eOld;
eOld = e;

== matlab function Subsystem3/Schema Motore 6/MATLAB Function ==
  data: e input double; u output double
function u = fcn(e)
persistent uOld;
persistent uOldOld;
persistent eOld;
persistent eOldOld;
if isempty(uOld)
   uOld = 0;
end
if isempty(uOldOld)
   uOldOld = 0;
end
if isempty(eOld)
   eOld = 0;
end
if isempty(eOldOld)
   eOldOld = 0;
end
%   9340 z^2 - 1.556e04 z + 6475    U(z)
%   ---------------------------- = ----
%        z^2 - 1.8 z + 0.8          E(z)
% U(z)*(z^2 - 1.8 z + 0.8) = E(z)*(9340 z^2 - 1.556e04 z + 6475)
% u(k+2)-1.8*u(k+1)+0.8*u(k)=9340*e(k+2)-1.556e04*e(k+1)+6475*e(k)
% u(k)-1.8*u(k-1)+0.8*u(k-1)=9340*e(k)-1.556e04*e(k-1)+6475*e(k-2)
% u(k)=1.8*u(k-1)-0.8*u(k-1)+9340*e(k)-1.556e04*e(k-1)+6475*e(k-2)
u = 1.8*uOld - 0.8*uOldOld + 9340*e - 15560*eOld + 6475*eOldOld;

uOldOld = uOld;
uOld = u;
eOldOld = eOld;
eOld = e;

== matlab function Subsystem3/Schema Motore 4/MATLAB Function ==
  data: e input double; u output double
function u = fcn(e)
persistent uOld;
persistent uOldOld;
persistent eOld;
persistent eOldOld;
if isempty(uOld)
   uOld = 0;
end
if isempty(uOldOld)
   uOldOld = 0;
end
if isempty(eOld)
   eOld = 0;
end
if isempty(eOldOld)
   eOldOld = 0;
end
%   9462 z^2 - 1.579e04 z + 6587    U(z)
%   ---------------------------- = -----
%        z^2 - 1.8 z + 0.8          E(z)
% U(z)*(z^2 - 1.8 z + 0.8) = E(z)*(9328 z^2 - 1.553e04 z + 6464)
u = 1.8*uOld - 0.8*uOldOld + 9462*e - 15790*eOld + 6587*eOldOld;

uOldOld = uOld;
uOld = u;
eOldOld = eOld;
eOld = e;
